simulink model "fs9_sim_sdr_dss"  (R2022b)
settings: Solver=ode4  StartTime=0.0  StopTime=duration  FixedStep=1/8  RelTol=1e-3
undefined symbols (not defined in the file or in its folder): Ke, Kv
settings Model: Creator=8049  LastModifiedBy=8049

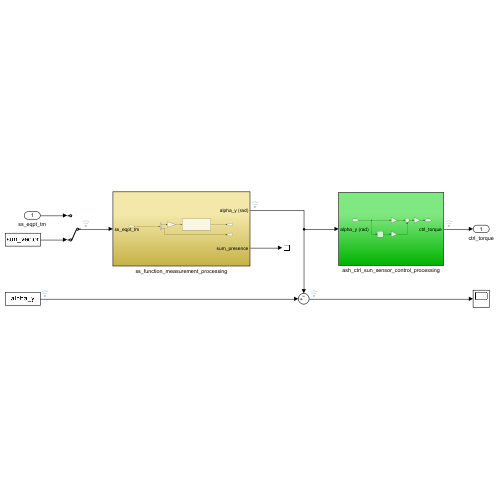
[thumbnail: Simulink's stored preview of the top-level diagram]
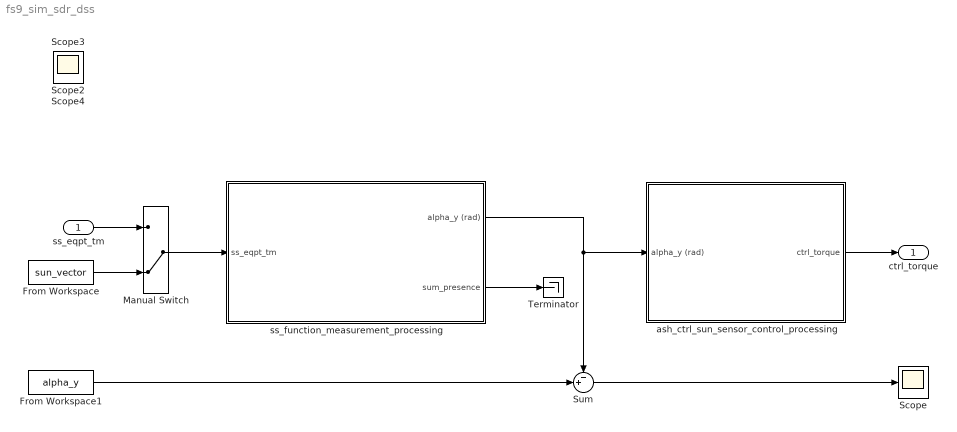
== system fs9_sim_sdr_dss ==
  ss_eqpt_tm : Inport
  From Workspace : FromWorkspace  VariableName=sun_vector
  From Workspace1 : FromWorkspace  VariableName=alpha_y
  Manual Switch : ManualSwitch  CurrentSetting=0
  Scope{,2..4} (4 alike) : Scope
  Sum : Sum  Inputs=-+|
  Terminator : Terminator
  ash_ctrl_sun_sensor_control_processing : Subsystem
  ss_function_measurement_processing : Subsystem
  ctrl_torque : Outport
  wires:
  Manual Switch/1 -> ss_function_measurement_processing/1(ss_eqpt_tm)
  ss_function_measurement_processing/1(alpha_y (rad)) -> ash_ctrl_sun_sensor_control_processing/1(alpha_y (rad)), Sum/1
  ash_ctrl_sun_sensor_control_processing/1(ctrl_torque) -> ctrl_torque/1
  ss_function_measurement_processing/2(sum_presence) -> Terminator/1
  ss_eqpt_tm/1 -> Manual Switch/1
  From Workspace1/1 -> Sum/2
  Sum/1 -> Scope/1
  From Workspace/1 -> Manual Switch/2

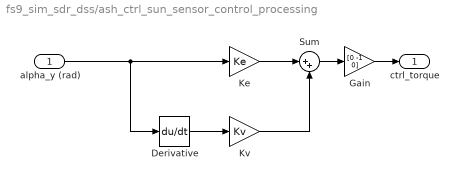
== system fs9_sim_sdr_dss/ash_ctrl_sun_sensor_control_processing ==
  alpha_y (rad) : Inport
  Derivative : Derivative
  Gain : Gain  Gain=[0 -1 0]
  Ke : Gain  Gain=Ke
  Kv : Gain  Gain=Kv
  Sum : Sum  Inputs=|++
  ctrl_torque : Outport
  wires:
  alpha_y (rad)/1 -> Derivative/1, Ke/1
  Derivative/1 -> Kv/1
  Ke/1 -> Sum/1
  Kv/1 -> Sum/2
  Sum/1 -> Gain/1
  Gain/1 -> ctrl_torque/1

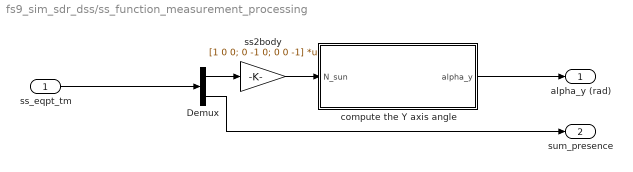
== system fs9_sim_sdr_dss/ss_function_measurement_processing ==
  ss_eqpt_tm : Inport
  Demux : Demux  Outputs=[3 1]
  compute the Y axis angle : MATLAB Function  TreatAsAtomicUnit=on
  ss2body : Gain  Gain=[1 0 0; 0 -1 0; 0 0 -1]  Multiplication=Matrix(K*u)
  alpha_y (rad) : Outport
  sum_presence : Outport  Port=2
  wires:
  compute the Y axis angle/1(alpha_y) -> alpha_y (rad)/1
  Demux/1 -> ss2body/1
  Demux/2 -> sum_presence/1
  ss_eqpt_tm/1 -> Demux/1
  ss2body/1 -> compute the Y axis angle/1(N_sun)

== matlab function fs9_sim_sdr_dss/ss_function_measurement_processing/compute the Y axis angle ==
  data: N_sun input; alpha_y output
function alpha_y = AlphaAngle(N_sun)
if norm(N_sun) > 0
    if sqrt(N_sun(3)^2+N_sun(1)^2) > 0
        alpha_y = acos(N_sun(3)/sqrt(N_sun(3)^2+N_sun(1)^2));
        if N_sun(1)>0
            alpha_y = alpha_y-pi;
        else
            alpha_y = pi-alpha_y;
        end
    else
        alpha_y = 0;
    end
else
    alpha_y = 0;
end
